simulink model "Greenhouse_4thPoint_PID"  (R2024a)
settings: Solver=VariableStepAuto  StartTime=0.0  StopTime=86400  RelTol=1e-3
values from neighbouring files (symbols this model uses):
  C_f1 = c_f * m_f1    (= 1846687500)    [init.m]
  C_f2 = c_f * m_f2    (= 492450000)    [init.m]
  kaf1 = t_t * Sm1_ext    (= 4731)    [init.m]
  kaf2 = t_t * Sm2_ext    (= 1311)    [init.m]
  kaf_int = t_t * Sm_int    (= 171)    [init.m]
  theta0_a = 100    [init.m]
  Ts = 1    [init.m]
  var_wf1 = 1    [init.m]
  var_wf2 = 1    [init.m]
undefined symbols (not defined in the file or in its folder): qMAX_m1, qMAX_m2, qmin_m1, qmin_m2
libraries: slpidlib x2
settings Model: Creator=loren  LastModifiedBy=leonardogiacobbe

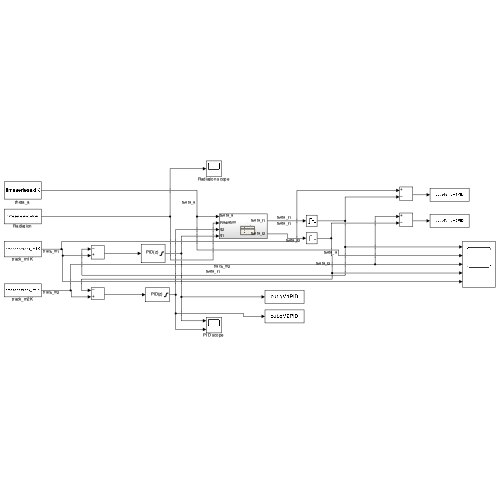
[thumbnail: Simulink's stored preview of the top-level diagram]
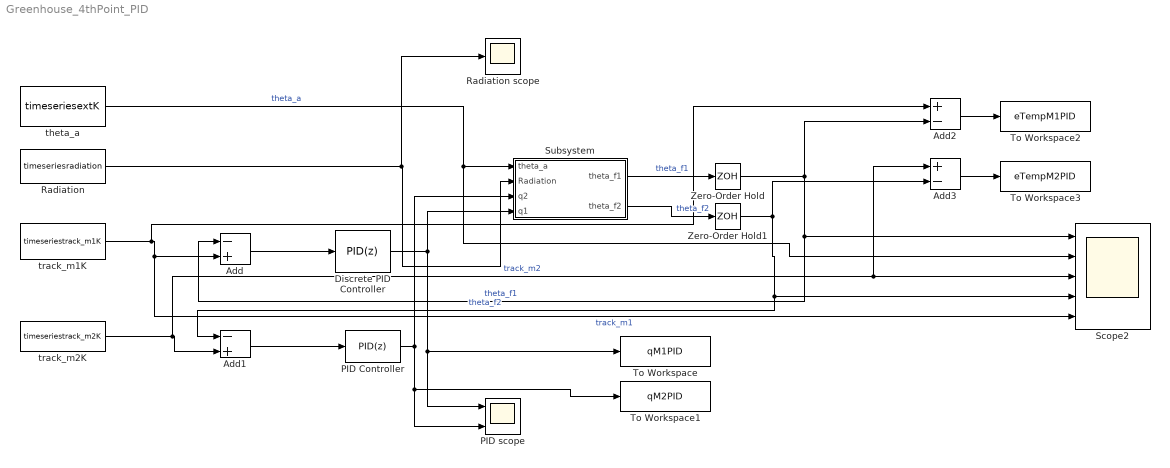
== system Greenhouse_4thPoint_PID ==
  Add : Sum  Inputs=-+
  Add1 : Sum  Inputs=-+
  Add2 : Sum  Inputs=+-
  Add3 : Sum  Inputs=+-
  Discrete PID Controller : slpidlib/PID Controller  Controller=PID  Form=Parallel  TimeDomain=Discrete-time  UseExternalTs=off  SampleTime=Ts  IntegratorMethod=Forward Euler  FilterMethod=Forward Euler  ControllerParametersSource=internal  P=183674446.5118  I=3575208.34127695  UseKiTs=off  D=-489865485.517858  UseExternalDerivativeSource=off  N=0.313161248470197  UseFilter=on  TunerSelectOption=Transfer Function Based (PID Tuner App)  InitialConditionSource=internal  InitialConditionForIntegrator=0  InitialConditionForFilter=0  DifferentiatorICPrevScaledInput=0  ExternalReset=none  TrackingMode=off  Kt=1  LimitOutput=on  SatLimitsSource=internal  UpperSaturationLimit=qMAX_m1  LowerSaturationLimit=qmin_m1  LinearizeAsGain=on  AntiWindupMode=none  Kb=1  LimitIntegrator=off  UpperIntegratorSaturationLimit=inf  LowerIntegratorSaturationLimit=-inf  POutMin=[]  POutMax=[]  IOutMin=[]  IOutMax=[]  DOutMin=[]  DOutMax=[]  NOutMin=[]  NOutMax=[]  SumOutMin=[]  SumOutMax=[]  SaturationOutMin=[]  SaturationOutMax=[]  PParamMin=[]  PParamMax=[]  IParamMin=[]  IParamMax=[]  DParamMin=[]  DParamMax=[]  NParamMin=[]  NParamMax=[]  KbParamMin=[]  KbParamMax=[]  KtParamMin=[]  KtParamMax=[]  KbOutMin=[]  KbOutMax=[]  KtOutMin=[]  KtOutMax=[]  IntegratorOutMin=[]  IntegratorOutMax=[]  FilterOutMin=[]  FilterOutMax=[]  SumI1OutMin=[]  SumI1OutMax=[]  SumI2OutMin=[]  SumI2OutMax=[]  SumI3OutMin=[]  SumI3OutMax=[]  SumI4OutMin=[]  SumI4OutMax=[]  SumDOutMin=[]  SumDOutMax=[]  DifferentiatorOutMin=[]  DifferentiatorOutMax=[]  FilterDiffOutCoefMin=[]  FilterDiffOutCoefMax=[]  ReciprocalOutMin=[]  ReciprocalOutMax=[]  SumDenOutMin=[]  SumDenOutMax=[]  SumNumOutMin=[]  SumNumOutMax=[]  DivideOutMin=[]  DivideOutMax=[]  UdiffTsProdOutMin=[]  UdiffTsProdOutMax=[]  NTsProdOutMin=[]  NTsProdOutMax=[]  UintegralTsProdOutMin=[]  UintegralTsProdOutMax=[]  UngainTsProdOutMin=[]  UngainTsProdOutMax=[]  ClampingZeroOutDataTypeStr=Inherit: Inherit via back propagation  ClampingZeroOutMin=[]  ClampingZeroOutMax=[]  FilterDenConstantOutDataTypeStr=Inherit: Inherit via back propagation  FilterDenConstantOutMin=[]  FilterDenConstantOutMax=[]  PCopyOutDataTypeStr=Inherit: Inherit via back propagation  PCopyOutMin=[]  PCopyOutMax=[]  NCopyOutDataTypeStr=Inherit: Inherit via back propagation  NCopyOutMin=[]  NCopyOutMax=[]  IntegratorContinuousStateAttributes=''  IntegratorStateMustResolveToSignalObject=off  IntegratorRTWStateStorageClass=Auto  FilterContinuousStateAttributes=''  FilterStateMustResolveToSignalObject=off  FilterRTWStateStorageClass=Auto  ParallelPVariant=InternalParameters  IdealPVariant=Disabled  IVariant=InternalParameters  DVariant=InternalParameters  IntegratorVariant=Discrete  SatVariant=Enabled  AWVariant=Passthrough  PCopyVariant=Disabled  TRVariant=Disabled  FdbkBlocksVariant=Forward  IdealPFdbkVariant=Disabled  SatFdbkVariant=Disabled  DerivativeFilterVariant=ForwardEulerFilter  NVariant=InternalParameters  NCopyVariant=Disabled  FilterICVariant=InternalICsFilter  IntegratorICVariant=InternalICs  ExternalResetVariant=Disabled  TRSumVariant=Passthrough  SumFdbkVariant=Disabled  SumVariant=Sum_PID  TsampFilterVariant=InternalTs  TsampNgainVariant=Passthrough  TsampIntegralVariant=Disabled_SignalSpec  ExternalSaturationOutDataTypeStr=Inherit: Same as second input  DerivativeSourceVariant=ErrorSignal
      settings: LibrarySourceBlock=simulink/Discrete/Discrete PID Controller
  PID Controller : slpidlib/PID Controller  Controller=PID  Form=Parallel  TimeDomain=Discrete-time  UseExternalTs=off  SampleTime=Ts  IntegratorMethod=Forward Euler  FilterMethod=Forward Euler  ControllerParametersSource=internal  P=14696921.5966059  I=86916.0087706669  UseKiTs=off  D=-130784547.359351  UseExternalDerivativeSource=off  N=0.106098963689464  UseFilter=on  TunerSelectOption=Transfer Function Based (PID Tuner App)  InitialConditionSource=internal  InitialConditionForIntegrator=0  InitialConditionForFilter=0  DifferentiatorICPrevScaledInput=0  ExternalReset=none  TrackingMode=off  Kt=1  LimitOutput=on  SatLimitsSource=internal  UpperSaturationLimit=qMAX_m2  LowerSaturationLimit=qmin_m2  LinearizeAsGain=on  AntiWindupMode=none  Kb=1  LimitIntegrator=off  UpperIntegratorSaturationLimit=inf  LowerIntegratorSaturationLimit=-inf  POutMin=[]  POutMax=[]  IOutMin=[]  IOutMax=[]  DOutMin=[]  DOutMax=[]  NOutMin=[]  NOutMax=[]  SumOutMin=[]  SumOutMax=[]  SaturationOutMin=[]  SaturationOutMax=[]  PParamMin=[]  PParamMax=[]  IParamMin=[]  IParamMax=[]  DParamMin=[]  DParamMax=[]  NParamMin=[]  NParamMax=[]  KbParamMin=[]  KbParamMax=[]  KtParamMin=[]  KtParamMax=[]  KbOutMin=[]  KbOutMax=[]  KtOutMin=[]  KtOutMax=[]  IntegratorOutMin=[]  IntegratorOutMax=[]  FilterOutMin=[]  FilterOutMax=[]  SumI1OutMin=[]  SumI1OutMax=[]  SumI2OutMin=[]  SumI2OutMax=[]  SumI3OutMin=[]  SumI3OutMax=[]  SumI4OutMin=[]  SumI4OutMax=[]  SumDOutMin=[]  SumDOutMax=[]  DifferentiatorOutMin=[]  DifferentiatorOutMax=[]  FilterDiffOutCoefMin=[]  FilterDiffOutCoefMax=[]  ReciprocalOutMin=[]  ReciprocalOutMax=[]  SumDenOutMin=[]  SumDenOutMax=[]  SumNumOutMin=[]  SumNumOutMax=[]  DivideOutMin=[]  DivideOutMax=[]  UdiffTsProdOutMin=[]  UdiffTsProdOutMax=[]  NTsProdOutMin=[]  NTsProdOutMax=[]  UintegralTsProdOutMin=[]  UintegralTsProdOutMax=[]  UngainTsProdOutMin=[]  UngainTsProdOutMax=[]  ClampingZeroOutDataTypeStr=Inherit: Inherit via back propagation  ClampingZeroOutMin=[]  ClampingZeroOutMax=[]  FilterDenConstantOutDataTypeStr=Inherit: Inherit via back propagation  FilterDenConstantOutMin=[]  FilterDenConstantOutMax=[]  PCopyOutDataTypeStr=Inherit: Inherit via back propagation  PCopyOutMin=[]  PCopyOutMax=[]  NCopyOutDataTypeStr=Inherit: Inherit via back propagation  NCopyOutMin=[]  NCopyOutMax=[]  IntegratorContinuousStateAttributes=''  IntegratorStateMustResolveToSignalObject=off  IntegratorRTWStateStorageClass=Auto  FilterContinuousStateAttributes=''  FilterStateMustResolveToSignalObject=off  FilterRTWStateStorageClass=Auto  ParallelPVariant=InternalParameters  IdealPVariant=Disabled  IVariant=InternalParameters  DVariant=InternalParameters  IntegratorVariant=Discrete  SatVariant=Enabled  AWVariant=Passthrough  PCopyVariant=Disabled  TRVariant=Disabled  FdbkBlocksVariant=Forward  IdealPFdbkVariant=Disabled  SatFdbkVariant=Disabled  DerivativeFilterVariant=ForwardEulerFilter  NVariant=InternalParameters  NCopyVariant=Disabled  FilterICVariant=InternalICsFilter  IntegratorICVariant=InternalICs  ExternalResetVariant=Disabled  TRSumVariant=Passthrough  SumFdbkVariant=Disabled  SumVariant=Sum_PID  TsampFilterVariant=InternalTs  TsampNgainVariant=Passthrough  TsampIntegralVariant=Disabled_SignalSpec  ExternalSaturationOutDataTypeStr=Inherit: Same as second input  DerivativeSourceVariant=ErrorSignal
  PID scope : Scope  NumInputPorts=2
  Radiation : FromWorkspace  VariableName=timeseriesradiation  SampleTime=Ts
  Radiation scope : Scope
  Scope2 : Scope  NumInputPorts=5
  Subsystem : Subsystem
  To Workspace : ToWorkspace  VariableName=qM1PID  SaveFormat=Timeseries  SampleTime=3600
  To Workspace1 : ToWorkspace  VariableName=qM2PID  SaveFormat=Timeseries  SampleTime=3600
  To Workspace2 : ToWorkspace  VariableName=eTempM1PID  SaveFormat=Timeseries  SampleTime=3600
  To Workspace3 : ToWorkspace  VariableName=eTempM2PID  SaveFormat=Timeseries  SampleTime=3600
  Zero-Order Hold : ZeroOrderHold  SampleTime=Ts
  Zero-Order Hold1 : ZeroOrderHold  SampleTime=Ts
  theta_a : FromWorkspace  VariableName=timeseriesextK  SampleTime=Ts
  track_m1K : FromWorkspace  VariableName=timeseriestrack_m1K  SampleTime=Ts
  track_m2K : FromWorkspace  VariableName=timeseriestrack_m2K  SampleTime=Ts
  wires:
  Subsystem/2(theta_f2) -> Zero-Order Hold1/1  "theta_f2"
  theta_a/1 -> Scope2/2, Subsystem/1(theta_a)  "theta_a"
  Zero-Order Hold1/1 -> Add1/1, Scope2/4, Add3/2  "theta_f2"
  Subsystem/1(theta_f1) -> Zero-Order Hold/1  "theta_f1"
  Radiation/1 -> Radiation scope/1, Subsystem/2(Radiation)
  track_m1K/1 -> Add2/1, Scope2/5, Add/2  "track_m1"
  Add/1 -> Discrete PID Controller/1
  Discrete PID Controller/1 -> Subsystem/4(q1), To Workspace/1, PID scope/1
  track_m2K/1 -> Add3/1, Scope2/3, Add1/2  "track_m2"
  Add1/1 -> PID Controller/1
  PID Controller/1 -> To Workspace1/1, PID scope/2, Subsystem/3(q2)
  Zero-Order Hold/1 -> Add2/2, Add/1, Scope2/1  "theta_f1"
  Add2/1 -> To Workspace2/1
  Add3/1 -> To Workspace3/1

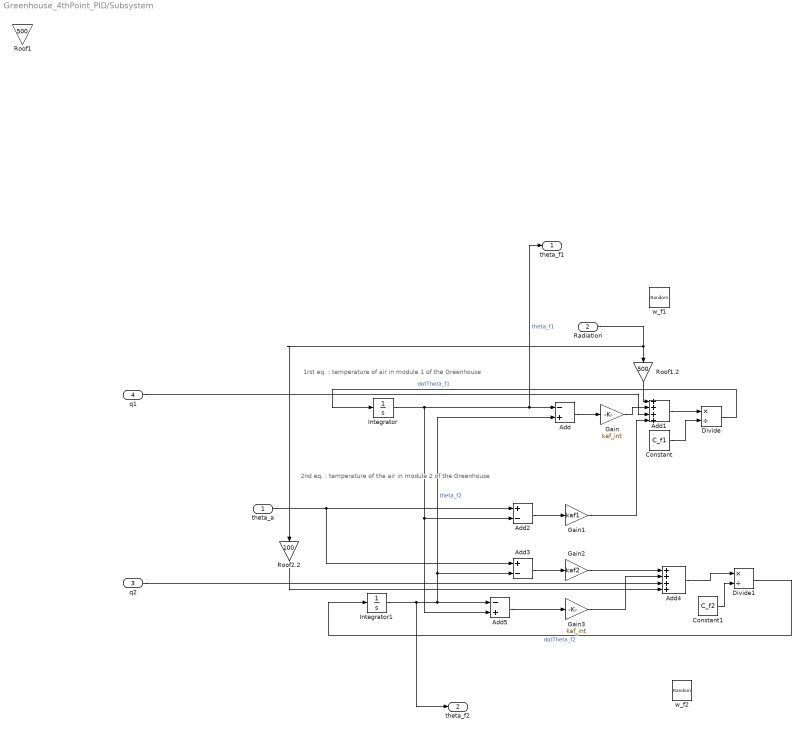
== system Greenhouse_4thPoint_PID/Subsystem ==
  note: 2nd eq. : temperature of the air in module 2 of the Greenhouse
  note: 1rst eq. : temperature of air in module 1 of the Greenhouse
  theta_a : Inport
  Radiation : Inport  Port=2
  q2 : Inport  Port=3
  q1 : Inport  Port=4
  Add : Sum  Inputs=-+
  Add1 : Sum  Inputs=++++
  Add2 : Sum  Inputs=+-
  Add3 : Sum  Inputs=+-
  Add4 : Sum  Inputs=++++
  Add5 : Sum  Inputs=-+
  Constant : Constant  Value=C_f1
  Constant1 : Constant  Value=C_f2
  Divide : Product  Inputs=*/
  Divide1 : Product  Inputs=*/
  Gain : Gain  Gain=kaf_int
  Gain1 : Gain  Gain=kaf1
  Gain2 : Gain  Gain=kaf2
  Gain3 : Gain  Gain=kaf_int
  Integrator : Integrator  InitialCondition=theta0_a
  Integrator1 : Integrator  InitialCondition=theta0_a
  Roof1 : Gain  Gain=500
  Roof1.2 : Gain  Gain=500
  Roof2.2 : Gain  Gain=100
  w_f1 : RandomNumber  Variance=var_wf1  SampleTime=Ts
  w_f2 : RandomNumber  Variance=var_wf2  SampleTime=Ts
  theta_f1 : Outport
  theta_f2 : Outport  Port=2
  wires:
  Add/1 -> Gain/1
  Gain1/1 -> Add1/4
  Add5/1 -> Gain3/1
  Add4/1 -> Divide1/1
  Integrator1/1 -> theta_f2/1, Add3/2, Add/2, Add5/1  "theta_f2"
  Divide1/1 -> Integrator1/1  "dotTheta_f2"
  Gain/1 -> Add1/2
  Radiation/1 -> Roof2.2/1, Roof1.2/1
  Constant/1 -> Divide/2
  Add1/1 -> Divide/1
  Add2/1 -> Gain1/1
  Add3/1 -> Gain2/1
  theta_a/1 -> Add3/1, Add2/1
  Integrator/1 -> Add5/2, Add2/2, theta_f1/1, Add/1  "theta_f1"
  Divide/1 -> Integrator/1  "dotTheta_f1"
  Gain3/1 -> Add4/2
  Gain2/1 -> Add4/1
  Constant1/1 -> Divide1/2
  Roof1.2/1 -> Add1/1
  Roof2.2/1 -> Add4/4
  q1/1 -> Add1/3
  q2/1 -> Add4/3
